simulink model "hdv_hydroelectropowertrain_model"  (R2023b)
settings: Solver=ode1be  StartTime=0.0  StopTime=simulation_length  FixedStep=tsample  MaxStep=tsample
values from neighbouring files (symbols this model uses):
  alpha = 35    [init_model.m]
  Apump = [0 1; 0 0]    [init_model.m]
  available_torque = torque_base+torque_friction_base    [init_model.m]
  Bpump = [0 1]'    [init_model.m]
  btheta_shaft = 2e2    (= 200)    [init_model.m]
  C1 = 10    [init_model.m]
  consumption = [consumption_1, consumption_2, consumption_3, consumption_4,          consumption_5, consumption_6, consumption_7, consumption_8,          consumption_9, consumption_10, consumption_11, consumption_12,          consumption_13, consumption_14, consumption_15, consumption_16          ]    [ic_engine_data.m]
  Cpump = [k 0]    [init_model.m]
  dp_lim = 400    [init_model.m]
  E0 = 3.685    [init_model.m]
  E1 = 0.2156    [init_model.m]
  E2 = 0    [init_model.m]
  E3 = 0    [init_model.m]
  E_1 = -1.031    [init_model.m]
  Elog = -0.05    [init_model.m]
  eta_v_m = 0.98    [init_model.m]
  eta_v_p = 0.97    [init_model.m]
  ki_dp_comp = 1/dp_lim    (= 0.0025)    [init_model.m]
  ki_te_comp = 2/te_lim    [init_model.m]
  kp_ctrl_m = 1    [init_model.m]
  kp_dp_comp = 0.5/dp_lim    (= 0.00125)    [init_model.m]
  kp_te_comp = 1/te_lim    [init_model.m]
  Kpump = acker(Apump,Bpump,poles)    [init_model.m]
  load_blade_enable = 0    [init_model.m]
  Lpump = acker(Apump',Cpump',pole_so)'    [init_model.m]
  M = 125    [init_model.m]
  Ncell = 185    [init_model.m]
  Npump = -1/(Cpump*inv(Apump-Bpump*Kpump)*Bpump)    [init_model.m]
  omega_e_rpm_ref = 1700    [init_model.m]
  omega_l_max_rpm = omega_l_max/(2*pi)*60    (= 50.3075969543)    [init_model.m]
  q1Kalman = tsample^2*1e-2    (= 1e-08)    [init_model.m]
  q2Kalman = tsample^1*1e-1    (= 0.0001)    [init_model.m]
  q3Kalman = 0    [init_model.m]
  Qhr = 400    [init_model.m]
  R0 = 0.015    [init_model.m]
  R1 = 0.015    [init_model.m]
  R_tg = 1.16/2    (= 0.58)    [init_model.m]
  rKalman = 1    [init_model.m]
  rpm_base = [620 700 800 900 1000 1100 1200 1300 1400 1500 1600 1700 1800      1900 2000 2100]    [ic_engine_data.m]
  rpm_consumption = rpm_base    [ic_engine_data.m]
  simulation_length = 245    [init_model.m]
  tau_load = 75e3    (= 75000)    [init_model.m]
  tau_load_max = 1600*41.4    (= 66240)    [init_model.m]
  Tc = tsample    (= 0.001)    [init_model.m]
  torque_base = [max(torque_16_data) max(torque_15_data) max(torque_14_data)      max(torque_13_data) max(torque_12_data) max(torque_11_data)      max(torque_10_data) max(torque_9_data) max(torque_8_data)      max(torque_7_data) max(torque_6_data) max(torque_5_data)      max(torque_4_data) max(torque_3_data) max(torque_2_data)      max(torque_1_data)]    [ic_engine_data.m]
  torque_consumption = torque_reference    [ic_engine_data.m]
  torque_friction_base = -(rpm_base./60*2*pi)*0.25-(rpm_base./60*2*pi).^2*5.2e-4    [ic_engine_data.m]
  tsample = 1e-3    (= 0.001)    [init_model.m]
  v_track1_ref = 8    [init_model.m]
  v_track2_ref = 8    [init_model.m]
  valve_mmorifice_max = 2.75    [init_model.m]
  xv_m_max = 1.2    [init_model.m]
undefined symbols (not defined in the file or in its folder): magnitude
libraries: fl_lib x381, nesl_utility x162, linear_swashplate_ctrl_lib x8, flexshaft_lib x5, bichamber_piston_lib x5, variable_displacement_motor_lib x4, variable_displacement_pump_lib x4, fixed_displacement_pump_lib x4, relief_valve_lib x4, inverse_shuttle_valve_lib x4, hydrostatic_threeway_valve_bichamber_piston_lib x4, hydrostatic_fourway_valve_bichamber_piston_lib x4
(part 9 of 9)

== system hdv_hydroelectropowertrain_model/PR776_powertrain/Hydrostatic_powertrain/driveline_RD2/vd_ctrl_pump_RD/servo pump RD ==
  displacement reference pu : Inport
  Gain : Gain  Gain=0.03647/2
  PS Gain : fl_lib/Physical Signals/Functions/PS Gain  gain=1/(0.03647/2) m^-1
  PS-Simulink Converter7 : nesl_utility/PS-Simulink Converter  PhysicalDomain=network_engine_domain  SubClassName=ps_output  LeftPortType=input  RightPortType=output  PseudoPeriodic=off  Frequencies=[]  VectorFormat=1-D array  Unit=1  AffineConversion=off
  hydrostatic_fourway_valve_bichamber : hydrostatic_fourway_valve_bichamber_piston_lib/hydrostatic_fourway_valve_bichamber  D1=D1 m  D2=D2 m  Lp=Lp m  xv_max=xv_max mm  mp=mp kg  kp=kp N/m  bp=bp N/(m/s)  q1_specify=off  q1_priority=None  q1=0 m^3/s  q1_nominal_specify=off  q1_nominal_unit=m^3/s  q1_nominal_value=1  q2_specify=off  q2_priority=None  q2=0 m^3/s  q2_nominal_specify=off  q2_nominal_unit=m^3/s  q2_nominal_value=1  qin_specify=off  qin_priority=None  qin=0 m^3/s  qin_nominal_specify=off  qin_nominal_unit=m^3/s  qin_nominal_value=1  qout_specify=off  qout_priority=None  qout=0 m^3/s  qout_nominal_specify=off  qout_nominal_unit=m^3/s  qout_nominal_value=1  p1_specify=off  p1_priority=High  p1=125 bar  p1_nominal_specify=off  p1_nominal_unit=bar  p1_nominal_value=1  p2_specify=off  p2_priority=High  p2=125 bar  p2_nominal_specify=off  p2_nominal_unit=bar  p2_nominal_value=1  fp_specify=off  fp_priority=None  fp=0 N  fp_nominal_specify=off  fp_nominal_unit=N  fp_nominal_value=1  vp_specify=off  vp_priority=None  vp=0 m/s  vp_nominal_specify=off  vp_nominal_unit=m/s  vp_nominal_value=1  xp_specify=off  xp_priority=High  xp=500 mm  xp_nominal_specify=off  xp_nominal_unit=mm  xp_nominal_value=1
      settings: InternalSimscapePortConfiguration="{\"Bottom\":[],\"Left\":[{\"id\":\"xv\",\"label\":\"xv\",\"type\":\"input\"},{\"id\":\"S\",\"label\":\"S\",\"type\":\"foundation.hydraulic.hydraulic\"},{\"id\":\"T\",\"label\":\"T\",\"type\":\"foundation.hydraulic.hydraulic\"}],\"Right\":[{\"id\":\"P\",\"label\":\"P\",\"type\":\"foundation.mechanical.translational.translational\"},{\"id\":\"xp_out\",\"label\":\"xp\",\"type\":\"output\"},{\"id\":\"q1_out\",\"label\":\"q1\",\"type\":\"output\"},{\"id\":\"q2_out\",\"label\":\"q2\",\"type\":\"output\"},{\"id\":\"p1_out\",\"label\":\"p1\",\"type\":\"output\"},{\"id\":\"p2_out\",\"label\":\"p2\",\"type\":\"output\"}],\"Top\":[]}"
  pmlinear_actuator : pm_linear_actuator_lib/pmlinear_actuator  Bm=1 s*V/m^2  mv=mv kg  Lc=Lc H  Rc=Rc Ohm  bv=bv N/(m/s)  h=h m  xv_max=xv_max mm  n=n  ic_specify=off  ic_priority=High  ic=0 A  ic_nominal_specify=off  ic_nominal_unit=A  ic_nominal_value=1  vv_specify=off  vv_priority=None  vv=0 m/s  vv_nominal_specify=off  vv_nominal_unit=m/s  vv_nominal_value=1  xv_specify=off  xv_priority=None  xv=0 m  xv_nominal_specify=off  xv_nominal_unit=m  xv_nominal_value=1
      settings: InternalSimscapePortConfiguration="{\"Bottom\":[],\"Left\":[{\"id\":\"uc\",\"label\":\"uc\",\"type\":\"input\"}],\"Right\":[{\"id\":\"xv_out\",\"label\":\"xv\",\"type\":\"output\"}],\"Top\":[]}"
  servo_ctrl : Subsystem
  pS : PMIOPort  Side=Left
  pT : PMIOPort  Port=2  Side=Left
  vd pu : PMIOPort  Port=3  Side=Right
  wires:
  displacement reference pu/1 -> Gain/1
  PS-Simulink Converter7/1 -> servo_ctrl/2(xp)  "xp"
  Gain/1 -> servo_ctrl/1(ref)
  connections:
  PS Gain/RConn1 -- vd pu/RConn1
  pmlinear_actuator/RConn1 -- hydrostatic_fourway_valve_bichamber/LConn1
  servo_ctrl/RConn1 -- pmlinear_actuator/LConn1
  PS-Simulink Converter7/LConn1 -- PS Gain/LConn1 -- hydrostatic_fourway_valve_bichamber/RConn2
  hydrostatic_fourway_valve_bichamber/LConn2 -- pS/RConn1
  hydrostatic_fourway_valve_bichamber/LConn3 -- pT/RConn1

== system hdv_hydroelectropowertrain_model/PR776_powertrain/electrical_main_drive_train/dc//dc/iin_ref/current_reference ==
  Constant1 : Constant  Value=250
  iin_ref : Outport
  wires:
  Constant1/1 -> iin_ref/1

== system hdv_hydroelectropowertrain_model/PR776_powertrain/electrical_main_drive_train/dc//dc/iout_ref/current_reference ==
  Constant1 : Constant  Value=350
  Manual Switch : ManualSwitch
  Rate Limiter2 : RateLimiter  RisingSlewLimit=500  FallingSlewLimit=-500  SampleTimeMode=inherited
  Step2 : Step  Time=simulation_length*3/5  Before=55e3/760  After=8e3/760  SampleTime=0
  Transfer Fcn1 : TransferFcn  Denominator=[1e-1 1]
  iout_ref : Outport
  wires:
  Step2/1 -> Rate Limiter2/1
  Rate Limiter2/1 -> Transfer Fcn1/1
  Constant1/1 -> Manual Switch/1
  Manual Switch/1 -> iout_ref/1
  Transfer Fcn1/1 -> Manual Switch/2

== system hdv_hydroelectropowertrain_model/PR776_powertrain/electrical_main_drive_train/dc//dc/vi ctrl/Iin Ctrl ==
  iin_ref : Inport
  iin : Inport  Port=2
  Sum2 : Sum  Inputs=+-  OutDataTypeStr=double  AccumDataTypeStr=double  SaturateOnIntegerOverflow=on
  iin_ctrl : Subsystem
  ctrli_out : Outport
  wires:
  Sum2/1 -> iin_ctrl/1(i_tilde)
  iin_ref/1 -> Sum2/1
  iin/1 -> Sum2/2
  iin_ctrl/1(ctrli_out) -> ctrli_out/1

== system hdv_hydroelectropowertrain_model/PR776_powertrain/electrical_main_drive_train/dc//dc/vi ctrl/Iout Ctrl ==
  iout_ref : Inport
  iout : Inport  Port=2
  Sum2 : Sum  Inputs=+-  OutDataTypeStr=double  AccumDataTypeStr=double  SaturateOnIntegerOverflow=on
  iout_ctrl : Subsystem
  ctrli_out : Outport
  wires:
  iout_ctrl/1(ctrli_out) -> ctrli_out/1
  iout/1 -> Sum2/2
  iout_ref/1 -> Sum2/1
  Sum2/1 -> iout_ctrl/1(i_tilde)

== system hdv_hydroelectropowertrain_model/PR776_powertrain/electrical_main_drive_train/dc//dc/vi ctrl/Vout Ctrl ==
  vout_ref : Inport
  vout : Inport  Port=2
  Sum2 : Sum  Inputs=+-  OutDataTypeStr=double  AccumDataTypeStr=double  SaturateOnIntegerOverflow=on
  vout_ctrl : Subsystem
  ctrlv_out : Outport
  wires:
  vout_ref/1 -> Sum2/1
  vout/1 -> Sum2/2
  vout_ctrl/1(ctrlv_out) -> ctrlv_out/1
  Sum2/1 -> vout_ctrl/1(ixi_tilde)

== system hdv_hydroelectropowertrain_model/PR776_powertrain/electrical_main_drive_train/dc//dc/vout_ref/voltage_reference ==
  Constant1 : Constant  Value=760
  vout_ref : Outport
  wires:
  Constant1/1 -> vout_ref/1

== system hdv_hydroelectropowertrain_model/PR776_powertrain/electrical_main_drive_train/pmsm_ctrl/pmsm_dq_ctrl/phaseU ==
  Controlled Current Source : fl_lib/Electrical/Electrical Sources/Controlled Current Source
  PS Divide : fl_lib/Physical Signals/Functions/PS Divide
  PS Saturation : fl_lib/Physical Signals/Nonlinear Operators/PS Saturation  upper_limit=inf V  lower_limit=1 V
  Resistor : fl_lib/Electrical/Electrical Elements/Resistor  R=1e4 Ohm  i_specify=off  i_priority=None  i=0 A  i_nominal_specify=off  i_nominal_unit=A  i_nominal_value=1  v_specify=off  v_priority=None  v=0 V  v_nominal_specify=off  v_nominal_unit=V  v_nominal_value=1
  Voltage Sensor : fl_lib/Electrical/Electrical Sensors/Voltage Sensor
  pin : PMIOPort  Side=Left
  u1+ : PMIOPort  Port=2  Side=Left
  u1- : PMIOPort  Port=3  Side=Left
  connections:
  pin/RConn1 -- PS Divide/LConn1
  Voltage Sensor/LConn1 -- Resistor/LConn1 -- u1+/RConn1 -- Controlled Current Source/RConn2
  PS Saturation/RConn1 -- PS Divide/LConn2
  Voltage Sensor/RConn2 -- Resistor/RConn1 -- u1-/RConn1 -- Controlled Current Source/LConn1
  Controlled Current Source/RConn1 -- PS Divide/RConn1
  Voltage Sensor/RConn1 -- PS Saturation/LConn1

== system hdv_hydroelectropowertrain_model/PR776_powertrain/front_blade_model/piston_tilt/controller/controller ==
  ref : Inport
  xp : Inport  Port=2
  Gain : Gain  Gain=200
  Saturation : Saturate  UpperLimit=valve_mmorifice_max  LowerLimit=-valve_mmorifice_max
  Simulink-PS Converter : nesl_utility/Simulink-PS Converter  PhysicalDomain=network_engine_domain  SubClassName=ps_input  LeftPortType=input  RightPortType=output  PseudoPeriodic=off  Frequencies=[]  NoiseDistribution=none  NoiseParameters=[]  Unit=mm  AffineConversion=on  FilteringAndDerivatives=provide  SimscapeFilterOrder=2  InputFilterTimeConstant=0.025  UdotUserProvided=0
  Sum3 : Sum  Inputs=-+|
  Unit Delay : UnitDelay  SampleTime=tsample  HasFrameUpgradeWarning=on
  Unit Delay1 : UnitDelay  SampleTime=tsample  HasFrameUpgradeWarning=on
  xv : PMIOPort  Side=Right
  wires:
  Unit Delay/1 -> Sum3/2
  xp/1 -> Unit Delay1/1
  Sum3/1 -> Gain/1
  Unit Delay1/1 -> Sum3/1
  Gain/1 -> Saturation/1
  ref/1 -> Unit Delay/1
  Saturation/1 -> Simulink-PS Converter/1
  connections:
  Simulink-PS Converter/RConn1 -- xv/RConn1

== system hdv_hydroelectropowertrain_model/PR776_powertrain/front_blade_model/pistons_height/controller/controller ==
  ref : Inport
  xp : Inport  Port=2
  Gain : Gain  Gain=200
  Saturation : Saturate  UpperLimit=valve_mmorifice_max  LowerLimit=-valve_mmorifice_max
  Simulink-PS Converter : nesl_utility/Simulink-PS Converter  PhysicalDomain=network_engine_domain  SubClassName=ps_input  LeftPortType=input  RightPortType=output  PseudoPeriodic=off  Frequencies=[]  NoiseDistribution=none  NoiseParameters=[]  Unit=mm  AffineConversion=on  FilteringAndDerivatives=provide  SimscapeFilterOrder=2  InputFilterTimeConstant=0.025  UdotUserProvided=0
  Sum3 : Sum  Inputs=-+|
  Unit Delay : UnitDelay  SampleTime=tsample  HasFrameUpgradeWarning=on
  Unit Delay1 : UnitDelay  SampleTime=tsample  HasFrameUpgradeWarning=on
  xv scope : Scope
  xv : PMIOPort  Side=Right
  wires:
  Sum3/1 -> Gain/1
  xp/1 -> Unit Delay1/1
  Unit Delay/1 -> Sum3/2
  Unit Delay1/1 -> Sum3/1
  ref/1 -> Unit Delay/1
  Gain/1 -> Saturation/1
  Saturation/1 -> xv scope/1, Simulink-PS Converter/1
  connections:
  Simulink-PS Converter/RConn1 -- xv/RConn1

== system hdv_hydroelectropowertrain_model/PR776_powertrain/front_blade_model/pistons_pitch/controller/controller ==
  ref : Inport
  xp : Inport  Port=2
  Gain : Gain  Gain=200
  Saturation : Saturate  UpperLimit=valve_mmorifice_max  LowerLimit=-valve_mmorifice_max
  Simulink-PS Converter : nesl_utility/Simulink-PS Converter  PhysicalDomain=network_engine_domain  SubClassName=ps_input  LeftPortType=input  RightPortType=output  PseudoPeriodic=off  Frequencies=[]  NoiseDistribution=none  NoiseParameters=[]  Unit=mm  AffineConversion=on  FilteringAndDerivatives=provide  SimscapeFilterOrder=2  InputFilterTimeConstant=0.025  UdotUserProvided=0
  Sum3 : Sum  Inputs=-+|
  Unit Delay : UnitDelay  SampleTime=tsample  HasFrameUpgradeWarning=on
  Unit Delay1 : UnitDelay  SampleTime=tsample  HasFrameUpgradeWarning=on
  xv : PMIOPort  Side=Right
  wires:
  Gain/1 -> Saturation/1
  Unit Delay1/1 -> Sum3/1
  Sum3/1 -> Gain/1
  xp/1 -> Unit Delay1/1
  Unit Delay/1 -> Sum3/2
  ref/1 -> Unit Delay/1
  Saturation/1 -> Simulink-PS Converter/1
  connections:
  Simulink-PS Converter/RConn1 -- xv/RConn1

== system hdv_hydroelectropowertrain_model/PR776_powertrain/Hydrostatic_powertrain/driveine_LD1/vd_ctrl_motor_LD/servo motor LD/servo_ctrl ==
  ref : Inport
  Constant : Constant
  Gain : Gain  Gain=0.06
  PS Gain : fl_lib/Physical Signals/Functions/PS Gain  gain=kp_ctrl_m
  PS Saturation : fl_lib/Physical Signals/Nonlinear Operators/PS Saturation  upper_limit=xv_m_max m  lower_limit=-xv_m_max m
  PS Subtract : fl_lib/Physical Signals/Functions/PS Subtract
  Simulink-PS Converter1 : nesl_utility/Simulink-PS Converter  PhysicalDomain=network_engine_domain  SubClassName=ps_input  LeftPortType=input  RightPortType=output  PseudoPeriodic=off  Frequencies=[]  NoiseDistribution=none  NoiseParameters=[]  Unit=m  AffineConversion=on  FilteringAndDerivatives=provide  SimscapeFilterOrder=2  InputFilterTimeConstant=0.025  UdotUserProvided=0
  Sum : Sum  Inputs=|-+
  xv : PMIOPort  Side=Right
  xp : PMIOPort  Port=2  Side=Left
  wires:
  Gain/1 -> Simulink-PS Converter1/1
  Sum/1 -> Gain/1
  Constant/1 -> Sum/2
  ref/1 -> Sum/1
  connections:
  PS Saturation/RConn1 -- xv/RConn1
  PS Saturation/LConn1 -- PS Gain/RConn1
  PS Gain/LConn1 -- PS Subtract/RConn1
  xp/RConn1 -- PS Subtract/LConn2
  PS Subtract/LConn1 -- Simulink-PS Converter1/RConn1

== system hdv_hydroelectropowertrain_model/PR776_powertrain/Hydrostatic_powertrain/driveine_LD1/vd_ctrl_pump_LD/servo pump RD/servo_ctrl ==
  ref : Inport
  xp : Inport  Port=2
  Gain : Gain  Gain=Bpump  Multiplication=Matrix(K*u)
  Gain1 : Gain  Gain=Apump  Multiplication=Matrix(K*u)
  Gain2 : Gain  Gain=Cpump  Multiplication=Matrix(K*u)
  Gain3 : Gain  Gain=Lpump  Multiplication=Matrix(K*u)
  Gain4 : Gain  Gain=Kpump  Multiplication=Matrix(K*u)
  Gain6 : Gain  Gain=Npump
  Integrator : Integrator
  Simulink-PS Converter1 : nesl_utility/Simulink-PS Converter  PhysicalDomain=network_engine_domain  SubClassName=ps_input  LeftPortType=input  RightPortType=output  PseudoPeriodic=off  Frequencies=[]  NoiseDistribution=none  NoiseParameters=[]  Unit=V  AffineConversion=off  FilteringAndDerivatives=provide  SimscapeFilterOrder=2  InputFilterTimeConstant=0.025  UdotUserProvided=0
  Sum : Sum  Inputs=|++
  Sum1 : Sum  Inputs=|++
  Sum2 : Sum  Inputs=+-|
  Sum3 : Sum  Inputs=-+|
  Transfer Fcn1 : TransferFcn  Denominator=[1e-6 1]
  uc : PMIOPort  Side=Right
  wires:
  Transfer Fcn1/1 -> Sum2/1
  Gain4/1 -> Sum3/1
  Gain6/1 -> Sum3/2
  ref/1 -> Gain6/1
  Integrator/1 -> Gain1/1, Gain2/1, Gain4/1
  Sum/1 -> Sum1/1
  Gain/1 -> Sum/1
  Gain1/1 -> Sum1/2
  Gain2/1 -> Sum2/2
  Sum2/1 -> Gain3/1
  xp/1 -> Transfer Fcn1/1
  Sum1/1 -> Integrator/1
  Gain3/1 -> Sum/2
  Sum3/1 -> Simulink-PS Converter1/1, Gain/1
  connections:
  uc/RConn1 -- Simulink-PS Converter1/RConn1

== system hdv_hydroelectropowertrain_model/PR776_powertrain/Hydrostatic_powertrain/driveine_LD2/vd_ctrl_motor_LD/servo motor LD/servo_ctrl ==
  ref : Inport
  Constant : Constant
  Gain : Gain  Gain=0.06
  PS Gain : fl_lib/Physical Signals/Functions/PS Gain  gain=kp_ctrl_m
  PS Saturation : fl_lib/Physical Signals/Nonlinear Operators/PS Saturation  upper_limit=xv_m_max m  lower_limit=-xv_m_max m
  PS Subtract : fl_lib/Physical Signals/Functions/PS Subtract
  Simulink-PS Converter1 : nesl_utility/Simulink-PS Converter  PhysicalDomain=network_engine_domain  SubClassName=ps_input  LeftPortType=input  RightPortType=output  PseudoPeriodic=off  Frequencies=[]  NoiseDistribution=none  NoiseParameters=[]  Unit=m  AffineConversion=on  FilteringAndDerivatives=provide  SimscapeFilterOrder=2  InputFilterTimeConstant=0.025  UdotUserProvided=0
  Sum : Sum  Inputs=|-+
  xv : PMIOPort  Side=Right
  xp : PMIOPort  Port=2  Side=Left
  wires:
  ref/1 -> Sum/1
  Constant/1 -> Sum/2
  Sum/1 -> Gain/1
  Gain/1 -> Simulink-PS Converter1/1
  connections:
  PS Subtract/LConn1 -- Simulink-PS Converter1/RConn1
  xp/RConn1 -- PS Subtract/LConn2
  PS Gain/LConn1 -- PS Subtract/RConn1
  PS Saturation/LConn1 -- PS Gain/RConn1
  PS Saturation/RConn1 -- xv/RConn1

== system hdv_hydroelectropowertrain_model/PR776_powertrain/Hydrostatic_powertrain/driveine_LD2/vd_ctrl_pump_LD/servo pump RD/servo_ctrl ==
  ref : Inport
  xp : Inport  Port=2
  Gain : Gain  Gain=Bpump  Multiplication=Matrix(K*u)
  Gain1 : Gain  Gain=Apump  Multiplication=Matrix(K*u)
  Gain2 : Gain  Gain=Cpump  Multiplication=Matrix(K*u)
  Gain3 : Gain  Gain=Lpump  Multiplication=Matrix(K*u)
  Gain4 : Gain  Gain=Kpump  Multiplication=Matrix(K*u)
  Gain6 : Gain  Gain=Npump
  Integrator : Integrator
  Simulink-PS Converter1 : nesl_utility/Simulink-PS Converter  PhysicalDomain=network_engine_domain  SubClassName=ps_input  LeftPortType=input  RightPortType=output  PseudoPeriodic=off  Frequencies=[]  NoiseDistribution=none  NoiseParameters=[]  Unit=V  AffineConversion=off  FilteringAndDerivatives=provide  SimscapeFilterOrder=2  InputFilterTimeConstant=0.025  UdotUserProvided=0
  Sum : Sum  Inputs=|++
  Sum1 : Sum  Inputs=|++
  Sum2 : Sum  Inputs=+-|
  Sum3 : Sum  Inputs=-+|
  Transfer Fcn1 : TransferFcn  Denominator=[1e-6 1]
  uc : PMIOPort  Side=Right
  wires:
  Sum3/1 -> Gain/1, Simulink-PS Converter1/1
  Gain3/1 -> Sum/2
  Sum1/1 -> Integrator/1
  xp/1 -> Transfer Fcn1/1
  Sum2/1 -> Gain3/1
  Gain2/1 -> Sum2/2
  Gain1/1 -> Sum1/2
  Gain/1 -> Sum/1
  Sum/1 -> Sum1/1
  Integrator/1 -> Gain4/1, Gain2/1, Gain1/1
  ref/1 -> Gain6/1
  Gain6/1 -> Sum3/2
  Gain4/1 -> Sum3/1
  Transfer Fcn1/1 -> Sum2/1
  connections:
  uc/RConn1 -- Simulink-PS Converter1/RConn1

== system hdv_hydroelectropowertrain_model/PR776_powertrain/Hydrostatic_powertrain/driveine_RD1/vd_ctrl_motor_RD/servo motor LD/servo_ctrl ==
  ref : Inport
  Constant : Constant
  Gain : Gain  Gain=0.06
  PS Gain : fl_lib/Physical Signals/Functions/PS Gain  gain=kp_ctrl_m
  PS Saturation : fl_lib/Physical Signals/Nonlinear Operators/PS Saturation  upper_limit=xv_m_max m  lower_limit=-xv_m_max m
  PS Subtract : fl_lib/Physical Signals/Functions/PS Subtract
  Simulink-PS Converter1 : nesl_utility/Simulink-PS Converter  PhysicalDomain=network_engine_domain  SubClassName=ps_input  LeftPortType=input  RightPortType=output  PseudoPeriodic=off  Frequencies=[]  NoiseDistribution=none  NoiseParameters=[]  Unit=m  AffineConversion=on  FilteringAndDerivatives=provide  SimscapeFilterOrder=2  InputFilterTimeConstant=0.025  UdotUserProvided=0
  Sum : Sum  Inputs=|-+
  xv : PMIOPort  Side=Right
  xp : PMIOPort  Port=2  Side=Left
  wires:
  ref/1 -> Sum/1
  Constant/1 -> Sum/2
  Sum/1 -> Gain/1
  Gain/1 -> Simulink-PS Converter1/1
  connections:
  PS Subtract/LConn1 -- Simulink-PS Converter1/RConn1
  xp/RConn1 -- PS Subtract/LConn2
  PS Gain/LConn1 -- PS Subtract/RConn1
  PS Saturation/LConn1 -- PS Gain/RConn1
  xv/RConn1 -- PS Saturation/RConn1

== system hdv_hydroelectropowertrain_model/PR776_powertrain/Hydrostatic_powertrain/driveine_RD1/vd_ctrl_pump_RD/servo pump RD/servo_ctrl ==
  ref : Inport
  xp : Inport  Port=2
  Gain : Gain  Gain=Bpump  Multiplication=Matrix(K*u)
  Gain1 : Gain  Gain=Apump  Multiplication=Matrix(K*u)
  Gain2 : Gain  Gain=Cpump  Multiplication=Matrix(K*u)
  Gain3 : Gain  Gain=Lpump  Multiplication=Matrix(K*u)
  Gain4 : Gain  Gain=Kpump  Multiplication=Matrix(K*u)
  Gain6 : Gain  Gain=Npump
  Integrator : Integrator
  Simulink-PS Converter1 : nesl_utility/Simulink-PS Converter  PhysicalDomain=network_engine_domain  SubClassName=ps_input  LeftPortType=input  RightPortType=output  PseudoPeriodic=off  Frequencies=[]  NoiseDistribution=none  NoiseParameters=[]  Unit=V  AffineConversion=off  FilteringAndDerivatives=provide  SimscapeFilterOrder=2  InputFilterTimeConstant=0.025  UdotUserProvided=0
  Sum : Sum  Inputs=|++
  Sum1 : Sum  Inputs=|++
  Sum2 : Sum  Inputs=+-|
  Sum3 : Sum  Inputs=-+|
  Transfer Fcn1 : TransferFcn  Denominator=[1e-6 1]
  uc : PMIOPort  Side=Right
  wires:
  Transfer Fcn1/1 -> Sum2/1
  Gain4/1 -> Sum3/1
  Gain6/1 -> Sum3/2
  ref/1 -> Gain6/1
  Integrator/1 -> Gain1/1, Gain2/1, Gain4/1
  Sum/1 -> Sum1/1
  Gain/1 -> Sum/1
  Gain1/1 -> Sum1/2
  Gain2/1 -> Sum2/2
  Sum2/1 -> Gain3/1
  xp/1 -> Transfer Fcn1/1
  Sum1/1 -> Integrator/1
  Gain3/1 -> Sum/2
  Sum3/1 -> Simulink-PS Converter1/1, Gain/1
  connections:
  uc/RConn1 -- Simulink-PS Converter1/RConn1

== system hdv_hydroelectropowertrain_model/PR776_powertrain/Hydrostatic_powertrain/driveline_RD2/vd_ctrl_motor_RD/servo motor LD/servo_ctrl ==
  ref : Inport
  Constant : Constant
  Gain : Gain  Gain=0.06
  PS Gain : fl_lib/Physical Signals/Functions/PS Gain  gain=kp_ctrl_m
  PS Saturation : fl_lib/Physical Signals/Nonlinear Operators/PS Saturation  upper_limit=xv_m_max m  lower_limit=-xv_m_max m
  PS Subtract : fl_lib/Physical Signals/Functions/PS Subtract
  Simulink-PS Converter1 : nesl_utility/Simulink-PS Converter  PhysicalDomain=network_engine_domain  SubClassName=ps_input  LeftPortType=input  RightPortType=output  PseudoPeriodic=off  Frequencies=[]  NoiseDistribution=none  NoiseParameters=[]  Unit=m  AffineConversion=on  FilteringAndDerivatives=provide  SimscapeFilterOrder=2  InputFilterTimeConstant=0.025  UdotUserProvided=0
  Sum : Sum  Inputs=|-+
  xv : PMIOPort  Side=Right
  xp : PMIOPort  Port=2  Side=Left
  wires:
  Gain/1 -> Simulink-PS Converter1/1
  Sum/1 -> Gain/1
  Constant/1 -> Sum/2
  ref/1 -> Sum/1
  connections:
  xv/RConn1 -- PS Saturation/RConn1
  PS Saturation/LConn1 -- PS Gain/RConn1
  PS Gain/LConn1 -- PS Subtract/RConn1
  xp/RConn1 -- PS Subtract/LConn2
  PS Subtract/LConn1 -- Simulink-PS Converter1/RConn1

== system hdv_hydroelectropowertrain_model/PR776_powertrain/Hydrostatic_powertrain/driveline_RD2/vd_ctrl_pump_RD/servo pump RD/servo_ctrl ==
  ref : Inport
  xp : Inport  Port=2
  Gain : Gain  Gain=Bpump  Multiplication=Matrix(K*u)
  Gain1 : Gain  Gain=Apump  Multiplication=Matrix(K*u)
  Gain2 : Gain  Gain=Cpump  Multiplication=Matrix(K*u)
  Gain3 : Gain  Gain=Lpump  Multiplication=Matrix(K*u)
  Gain4 : Gain  Gain=Kpump  Multiplication=Matrix(K*u)
  Gain6 : Gain  Gain=Npump
  Integrator : Integrator
  Simulink-PS Converter1 : nesl_utility/Simulink-PS Converter  PhysicalDomain=network_engine_domain  SubClassName=ps_input  LeftPortType=input  RightPortType=output  PseudoPeriodic=off  Frequencies=[]  NoiseDistribution=none  NoiseParameters=[]  Unit=V  AffineConversion=off  FilteringAndDerivatives=provide  SimscapeFilterOrder=2  InputFilterTimeConstant=0.025  UdotUserProvided=0
  Sum : Sum  Inputs=|++
  Sum1 : Sum  Inputs=|++
  Sum2 : Sum  Inputs=+-|
  Sum3 : Sum  Inputs=-+|
  Transfer Fcn1 : TransferFcn  Denominator=[1e-6 1]
  uc : PMIOPort  Side=Right
  wires:
  Sum3/1 -> Gain/1, Simulink-PS Converter1/1
  Gain3/1 -> Sum/2
  Sum1/1 -> Integrator/1
  xp/1 -> Transfer Fcn1/1
  Sum2/1 -> Gain3/1
  Gain2/1 -> Sum2/2
  Gain1/1 -> Sum1/2
  Gain/1 -> Sum/1
  Sum/1 -> Sum1/1
  Integrator/1 -> Gain4/1, Gain2/1, Gain1/1
  ref/1 -> Gain6/1
  Gain6/1 -> Sum3/2
  Gain4/1 -> Sum3/1
  Transfer Fcn1/1 -> Sum2/1
  connections:
  uc/RConn1 -- Simulink-PS Converter1/RConn1

== system hdv_hydroelectropowertrain_model/PR776_powertrain/electrical_main_drive_train/dc//dc/vi ctrl/Iin Ctrl/iin_ctrl ==
  i_tilde : Inport
  1/Ti : Gain  Gain=0.25  ParamDataTypeStr=double  OutDataTypeStr=double  SaturateOnIntegerOverflow=on
  1/Ti1 : Gain  ParamDataTypeStr=double  OutDataTypeStr=double  SaturateOnIntegerOverflow=on
  Saturation2 : Saturate  UpperLimit=12  LowerLimit=0  OutDataTypeStr=double
  Sum1 : Sum  Inputs=+++  SaturateOnIntegerOverflow=on
  Sum4 : Sum  Inputs=-+  SaturateOnIntegerOverflow=on
  Unit Delay4 : UnitDelay  SampleTime=tsample  HasFrameUpgradeWarning=on
  kp2 : Gain  Gain=18*tsample  ParamDataTypeStr=double  OutDataTypeStr=double  SaturateOnIntegerOverflow=on
  ctrli_out : Outport
  wires:
  1/Ti1/1 -> 1/Ti/1, kp2/1
  Saturation2/1 -> ctrli_out/1, Sum4/2
  Unit Delay4/1 -> Sum1/3
  Sum4/1 -> Unit Delay4/1
  1/Ti/1 -> Sum4/1, Sum1/1
  kp2/1 -> Sum1/2
  Sum1/1 -> Saturation2/1
  i_tilde/1 -> 1/Ti1/1

== system hdv_hydroelectropowertrain_model/PR776_powertrain/electrical_main_drive_train/dc//dc/vi ctrl/Iout Ctrl/iout_ctrl ==
  i_tilde : Inport
  1/Ti : Gain  Gain=0.25  ParamDataTypeStr=double  OutDataTypeStr=double  SaturateOnIntegerOverflow=on
  1/Ti1 : Gain  ParamDataTypeStr=double  OutDataTypeStr=double  SaturateOnIntegerOverflow=on
  Saturation2 : Saturate  UpperLimit=12  LowerLimit=0  OutDataTypeStr=double
  Sum1 : Sum  Inputs=+++  SaturateOnIntegerOverflow=on
  Sum4 : Sum  Inputs=-+  SaturateOnIntegerOverflow=on
  Unit Delay4 : UnitDelay  SampleTime=tsample  HasFrameUpgradeWarning=on
  kp2 : Gain  Gain=18*tsample  ParamDataTypeStr=double  OutDataTypeStr=double  SaturateOnIntegerOverflow=on
  ctrli_out : Outport
  wires:
  i_tilde/1 -> 1/Ti1/1
  Sum1/1 -> Saturation2/1
  kp2/1 -> Sum1/2
  1/Ti/1 -> Sum1/1, Sum4/1
  Sum4/1 -> Unit Delay4/1
  Unit Delay4/1 -> Sum1/3
  Saturation2/1 -> Sum4/2, ctrli_out/1
  1/Ti1/1 -> kp2/1, 1/Ti/1

== system hdv_hydroelectropowertrain_model/PR776_powertrain/electrical_main_drive_train/dc//dc/vi ctrl/Vout Ctrl/vout_ctrl ==
  ixi_tilde : Inport
  1/Ti : Gain  Gain=0.25  ParamDataTypeStr=double  OutDataTypeStr=double  SaturateOnIntegerOverflow=on
  1/Ti1 : Gain  ParamDataTypeStr=double  OutDataTypeStr=double  SaturateOnIntegerOverflow=on
  Saturation2 : Saturate  UpperLimit=12  LowerLimit=0  OutDataTypeStr=double
  Sum1 : Sum  Inputs=+++  SaturateOnIntegerOverflow=on
  Sum4 : Sum  Inputs=-+  SaturateOnIntegerOverflow=on
  Unit Delay4 : UnitDelay  SampleTime=tsample  HasFrameUpgradeWarning=on
  kp2 : Gain  Gain=18*tsample  ParamDataTypeStr=double  OutDataTypeStr=double  SaturateOnIntegerOverflow=on
  ctrlv_out : Outport
  wires:
  ixi_tilde/1 -> 1/Ti1/1
  kp2/1 -> Sum1/2
  Sum4/1 -> Unit Delay4/1
  1/Ti/1 -> Sum1/1, Sum4/1
  Sum1/1 -> Saturation2/1
  Unit Delay4/1 -> Sum1/3
  Saturation2/1 -> ctrlv_out/1, Sum4/2
  1/Ti1/1 -> 1/Ti/1, kp2/1

== matlab function hdv_hydroelectropowertrain_model/PR776_powertrain/electrical_main_drive_train/battery_management/kalman_observer_gains ==
  data: iz input; ts input; l1 output; z input; q1 input; q2 input; q3 input; r input; Qhr input; l2 output; l3 output
function [l1,l2,l3] = EKF(iz,ts,z,q1,q2,q3,r,Qhr)

    persistent  p11 p12 p13 p21 p22 p23 p31 p32 p33

    if isempty(p11)
        p11 = q1;
        p12 = 0;
        p13 = 0;
        p21 = 0;
        p22 = q2;
        p23 = 0;
        p31 = 0;
        p32 = 0;
        p33 = q3;
    end
    R = 0.015;
    C = 10;
    M = 125;
    E_1 = -1.031;
    E1 = 0.2156;
    E2 = 0;
    E3 = 0;
    Elog = -0.05;
    alpha = 35;
    Q = Qhr*3600;

    a11 = 1;
    a12 = 0;
    a13 = 0;
    a21 = 0;
    a22 = exp(-ts/(R*C));
    a23 = 0;
    a31 = 0;
    a32 = 0;
    a33 = abs(exp(-iz*ts/Q));

    c1 = -alpha*E_1*abs(exp(-alpha*z)) + E1 + 2*E2*z + 3*E3*z^2 - Elog/(1-z+ts);
    c2 = -R;
    c3 = M;
    
    p11_pr = a11*(a11*p11 + a12*p21 + a13*p31) + a12*(a11*p12 + a12*p22 + a13*p32) + a13*(a11*p13 + a12*p23 + a13*p33) + q1;

    p12_pr = a21*(a11*p11 + a12*p21 + a13*p31) + a22*(a11*p12 + a12*p22 + a13*p32) + a23*(a11*p13 + a12*p23 + a13*p33);

    p13_pr = a31*(a11*p11 + a12*p21 + a13*p31) + a32*(a11*p12 + a12*p22 + a13*p32) + a33*(a11*p13 + a12*p23 + a13*p33);

    p21_pr = a11*(a21*p11 + a22*p21 + a23*p31) + a12*(a21*p12 + a22*p22 + a23*p32) + a13*(a21*p13 + a22*p23 + a23*p33);

    p22_pr = a21*(a21*p11 + a22*p21 + a23*p31) + a22*(a21*p12 + a22*p22 + a23*p32) + a23*(a21*p13 + a22*p23 + a23*p33) + q2;

    p23_pr = a31*(a21*p11 + a22*p21 + a23*p31) + a32*(a21*p12 + a22*p22 + a23*p32) + a33*(a21*p13 + a22*p23 + a23*p33);

    p31_pr = a11*(a31*p11 + a32*p21 + a33*p31) + a12*(a31*p12 + a32*p22 + a33*p32) + a13*(a31*p13 + a32*p23 + a33*p33);

    p32_pr = a21*(a31*p11 + a32*p21 + a33*p31) + a22*(a31*p12 + a32*p22 + a33*p32) + a23*(a31*p13 + a32*p23 + a33*p33);

    p33_pr = a31*(a31*p11 + a32*p21 + a33*p31) + a32*(a31*p12 + a32*p22 + a33*p32) + a33*(a31*p13 + a32*p23 + a33*p33) + q3;

    den = c1*(c1*p11 + c2*p21 + c3*p31) + c2*(c1*p12 + c2*p22 + c3*p32) + c3*(c1*p13 + c2*p23 + c3*p33) + r;
 
    l1 = (c1*p11 + c2*p12 + c3*p13)/den;
    l2 = (c1*p21 + c2*p22 + c3*p23)/den;
    l3 = (c1*p31 + c2*p32 + c3*p33)/den;
    
    p11 = (1 - c1*l1)*p11_pr - c2*l1*p21_pr - c3*l1*p31_pr;
    
    p12 = (1 - c1*l1)*p12_pr - c2*l1*p22_pr - c3*l1*p32_pr;
    
    p13 = (1 - c1*l1)*p13_pr - c2*l1*p23_pr - c3*l1*p33_pr;
    
    p21 = -c1*l2*p11_pr + (1 - c2*l2)*p21_pr - c3*l2*p31_pr;
    
    p22 = -c1*l2*p12_pr + (1 - c2*l2)*p22_pr - c3*l2*p32_pr;
    
    p23 = -c1*l2*p13_pr + (1 - c2*l2)*p23_pr - c3*l2*p33_pr;
    
    p31 = -c1*l3*p11_pr - c2*l3*p21_pr + (1 - c3*l3)*p31_pr;
    
    p32 = -c1*l3*p12_pr - c2*l3*p22_pr + (1 - c3*l3)*p32_pr;
    
    p33 = -c1*l3*p13_pr - c2*l3*p23_pr + (1 - c3*l3)*p33_pr;
end

== matlab function hdv_hydroelectropowertrain_model/Vehicle Control System/feedforwards/Volumetric displacements calculation ==
  data: omega_e_rpm_ref input; Vd_p_R output; v_track1_ref input; v_track2_ref input; eta_vol_pump_right input; eta_vol_pump_left input; eta_vol_motor_right input; eta_vol_motor_left input; Vd_p_L output; v_track1_ref_cond output; v_track2_ref_cond output
function [Vd_p_R, Vd_p_L, v_track1_ref_cond, v_track2_ref_cond] = fcn(omega_e_rpm_ref, v_track1_ref, v_track2_ref, eta_vol_pump_right, eta_vol_pump_left, eta_vol_motor_right, eta_vol_motor_left)

n_tg = 54.31;
R_tg = 1.16/2;
Vm_nom = 280*2;
Vp_nom = 210*2;
v_track_sum_max = 18;
v_track_diff_max = 4;

eta_vol_tot_right = eta_vol_pump_right*eta_vol_motor_right;
eta_vol_tot_left = eta_vol_pump_left*eta_vol_motor_left;

v_track_sum = v_track1_ref + v_track2_ref;
v_track_diff = v_track1_ref - v_track2_ref;

if v_track_sum >= v_track_sum_max
    v_track_sum = v_track_sum_max;
end

if v_track_sum <= -v_track_sum_max
    v_track_sum = -v_track_sum_max;
end

if v_track_diff >= v_track_diff_max
    v_track_diff = v_track_diff_max;
end

if v_track_diff <= -v_track_diff_max
    v_track_diff = -v_track_diff_max;
end

v_track1_ref_cond = 1/2*(v_track_sum + v_track_diff);
v_track2_ref_cond = 1/2*(v_track_sum - v_track_diff);

omega_l_1_ref_rpm = v_track1_ref_cond/3.6/R_tg/(2*pi)*60;
omega_l_2_ref_rpm = v_track2_ref_cond/3.6/R_tg/(2*pi)*60;

d1_ff_temp = abs(Vm_nom/Vp_nom/eta_vol_tot_right*omega_l_1_ref_rpm/omega_e_rpm_ref*n_tg);
d2_ff_temp = abs(Vm_nom/Vp_nom/eta_vol_tot_left*omega_l_2_ref_rpm/omega_e_rpm_ref*n_tg);

if d1_ff_temp >= 1
    Vd_p_R = 2 - 1/d1_ff_temp;
else
    Vd_p_R = d1_ff_temp;
end
if d2_ff_temp >= 1
    Vd_p_L = 2 - 1/d2_ff_temp;
else
    Vd_p_L = d2_ff_temp;
end

== matlab function hdv_hydroelectropowertrain_model/PR776_powertrain/electrical_main_drive_train/battery_management/lithium-ion battery model ==
  data: iz input; SOC output; u output; ts input; Qhr input; l1 input; l2 input; l3 input; vout input; x output
function [SOC, u, x] = lithium_ion_battery(iz,ts,Qhr,l1,l2,l3,vout)

    persistent z_po ir_po h_po vout_hat

    if isempty(z_po)
        ir_po = 0;
        h_po = 0;
        z_po = 0;        
    end
    
        R0 = 0.015;
        R = 0.015;
        C = 10;
        M = 125;
        E_1 = -1.031;
        E0 = 3.685;
        E1 = 0.2156;
        E2 = 0;
        E3 = 0;
        Elog = -0.05;
        alpha = 35;
        N = 185;
        Q = Qhr*3600;
        
        
        if z_po > 1
            z_pr = z_po;
        elseif z_po < 0
            z_pr = z_po;
        else
            z_pr = z_po - ts/Q*iz ;
        end
        ir_pr = exp(-ts/(R*C))*ir_po + (1-exp(-ts/(R*C)))*iz;

        h_pr = exp(-abs(iz)*ts/Q)*h_po - (1-exp(-abs(iz)*ts/Q))*sign(iz);
        
        OCV = E_1*exp(-z_pr*alpha) + E0 + E1*z_pr + E2*z_pr^2 + E3*z_pr^3 + Elog * log(abs(1-z_pr+ts));
        
        vout_hat = OCV*N + M*h_pr - R*ir_pr - R0*iz;
        
        z_po = z_pr + l1*(vout - vout_hat);
        ir_po = ir_pr + l2*(vout - vout_hat);
        h_po = h_pr + l3*(vout - vout_hat);
        u = vout_hat;
        
        x = [z_po; ir_po; h_po];

    SOC = z_po;
end
